simulink model "OutputToVisualizationAveragedEEG"  (R2016b)
settings: Solver=FixedStepDiscrete  StartTime=0.0  StopTime=10.0  FixedStep=sCoreParams.core.stepPeriod  RelTol=1e-3  EnableMultiTasking=on
undefined symbols (not defined in the file or in its folder): sCoreParams, sCoreParams_viz_channelInds
libraries: dspindex x3, slrtlib x2, xpcrtudplib x2, xpcutilitieslib x1, xpcobsoletelib x1
settings Model: DataTypeOverride=Double  MinMaxOverflowLogging=ForceOff  Creator=rzelmann  LastModifiedBy=Rina
settings SolverCC: EnableConcurrentExecution=on  ConcurrentTasks=on  AutoInsertRateTranBlk=on
settings DataIOCC: SaveFormat=StructureWithTime  SaveOutput=off  SignalLogging=off  DSMLogging=off  SaveTime=off
settings OptimizationCC: BlockReduction=off  DefaultParameterBehavior=Inlined  LifeSpan=inf
settings DebuggingCC: AllowSymbolicDim=off  SFUnexpectedBacktrackingDiag=warning  SFNoUnconditionalDefaultTransitionDiag=warning  SFExecutionAtInitializationDiag=none
settings HardwareCC: ProdBitPerPointer=32  ProdBitPerSizeT=32  ProdBitPerPtrDiffT=32  ProdLargestAtomicFloat=None  ProdWordSize=32  ProdLongLongMode=on  ProdHWDeviceType=Generic->32-bit x86 compatible
settings ModelReferenceCC: UpdateModelReferenceTargets=Force  ParallelModelReferenceMATLABWorkerInit=Load Top Model  ModelReferenceNumInstancesAllowed=Single  ModelReferencePassRootInputsByReference=off
settings RTWCC: SystemTargetFile=slrt.tlc  TemplateMakefile=slrt_default_tmf  Description=Simulink Real-Time  RTWCompilerOptimization=on
settings CodeAppCC: MaxIdLength=63
settings TargetCC: CodeReplacementLibrary=XPC_BLAS  ParMdlRefBuildCompliant=on  ConcurrentExecutionCompliant=on  GeneratePreprocessorConditionals=Use local settings  MatFileLogging=on  MATLABClassNameForMDSCustomization=xpcAperiodicCustomization
settings ConfigComp: CovMetricSettings=dw  CovHtmlReporting=on  CovSaveCumulativeToWorkspaceVar=on  CovSaveSingleToWorkspaceVar=on  CovExternalEMLEnable=off

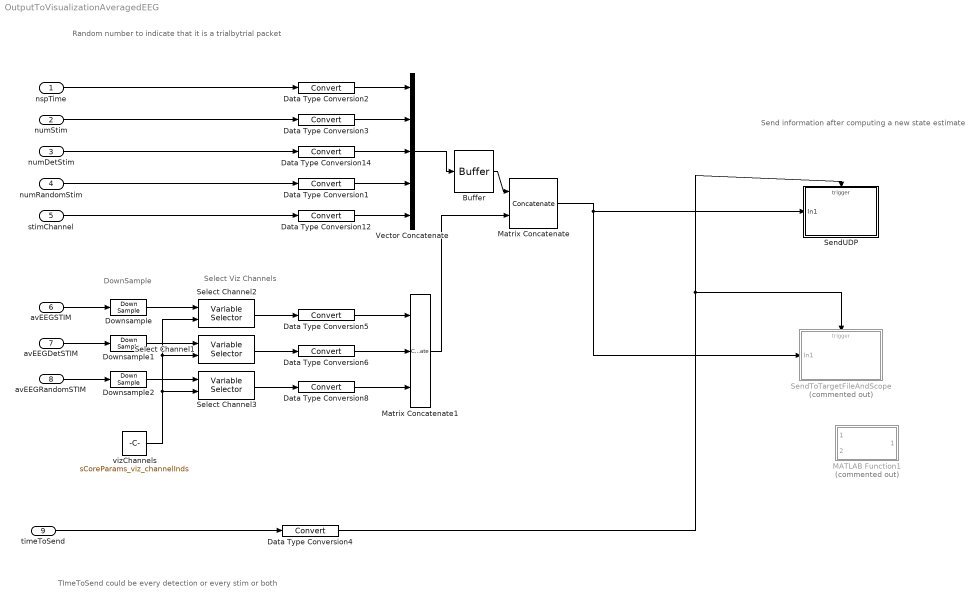
== system OutputToVisualizationAveragedEEG ==
  note: Select Viz Channels
  note: DownSample
  note: TImeToSend could be every detection or every stim or both
  note: Random number to indicate that it is a trialbytrial packet
  note: Send information after computing a new state estimate
  nspTime : Inport  PortDimensions=1  SampleTime=sCoreParams.core.stepPeriod
  numStim : Inport  Port=2  OutDataTypeStr=double  PortDimensions=1  SampleTime=sCoreParams.core.stepPeriod
  numDetStim : Inport  Port=3  OutDataTypeStr=double  PortDimensions=1  SampleTime=sCoreParams.core.stepPeriod
  numRandomStim : Inport  Port=4  PortDimensions=1  SampleTime=sCoreParams.core.stepPeriod
  stimChannel : Inport  Port=5  OutDataTypeStr=int32  PortDimensions=[1 2]  SampleTime=sCoreParams.core.stepPeriod  Interpolate=off
  avEEGSTIM : Inport  Port=6  PortDimensions=[sCoreParams.viz.DurationTriggerAvSamp sCoreParams.decoders.txDetector.nChannels]  SampleTime=sCoreParams.core.stepPeriod
  avEEGDetSTIM : Inport  Port=7  PortDimensions=[sCoreParams.viz.DurationTriggerAvSamp sCoreParams.decoders.txDetector.nChannels]  SampleTime=sCoreParams.core.stepPeriod
  avEEGRandomSTIM : Inport  Port=8  PortDimensions=[sCoreParams.viz.DurationTriggerAvSamp sCoreParams.decoders.txDetector.nChannels]  SampleTime=sCoreParams.core.stepPeriod
  timeToSend : Inport  Port=9  OutDataTypeStr=boolean  PortDimensions=1  SampleTime=sCoreParams.core.stepPeriod
  Buffer : Buffer  N=sCoreParams.write.broadcastAvEEGSamp  V=sCoreParams.write.broadcastAvEEGSamp-1  TreatMby1Signals=One channel  OutputFrames=off
  Data Type Conversion{1..6,8,12,14} (9 alike) : DataTypeConversion
  Downsample : DownSample  N=sCoreParams.write.averagedEEGDownSampling
  Downsample1 : DownSample  N=sCoreParams.write.averagedEEGDownSampling
  Downsample2 : DownSample  N=sCoreParams.write.averagedEEGDownSampling
  MATLAB Function1 : MATLAB Function  Commented=on  TreatAsAtomicUnit=on
  Matrix Concatenate : Concatenate  Mode=Multidimensional array  ConcatenateDimension=2
  Matrix Concatenate1 : Concatenate  NumInputs=3  Mode=Multidimensional array  ConcatenateDimension=2
  Select Channel1 : dspindex/Variable Selector  NumInputs=1  rowsOrCols=Columns  IdxMode=Variable  Elements=sCoreParams_decoders_txDetector_channel1  ZerOneIdxMode=One-based  errmode=Clip Index  FillMode=off  FillValues=0
  Select Channel2 : dspindex/Variable Selector  NumInputs=1  rowsOrCols=Columns  IdxMode=Variable  Elements=sCoreParams_decoders_txDetector_channel1  ZerOneIdxMode=One-based  errmode=Clip Index  FillMode=off  FillValues=0
  Select Channel3 : dspindex/Variable Selector  NumInputs=1  rowsOrCols=Columns  IdxMode=Variable  Elements=sCoreParams_decoders_txDetector_channel1  ZerOneIdxMode=One-based  errmode=Clip Index  FillMode=off  FillValues=0
  SendToTargetFileAndScope : Subsystem  Commented=on
  SendUDP : Subsystem
  Vector Concatenate : Concatenate  NumInputs=5
  vizChannels : Constant  Value=sCoreParams_viz_channelInds
  wires:
  avEEGDetSTIM/1 -> Downsample1/1
  Data Type Conversion2/1 -> Vector Concatenate/1
  Select Channel1/1 -> Data Type Conversion6/1
  Vector Concatenate/1 -> Buffer/1
  Matrix Concatenate1/1 -> Matrix Concatenate/2
  Matrix Concatenate/1 -> SendToTargetFileAndScope/1(In1), SendUDP/1(In1)
  stimChannel/1 -> Data Type Conversion12/1
  nspTime/1 -> Data Type Conversion2/1
  numStim/1 -> Data Type Conversion3/1
  avEEGSTIM/1 -> Downsample/1
  numRandomStim/1 -> Data Type Conversion1/1
  Data Type Conversion5/1 -> Matrix Concatenate1/1
  numDetStim/1 -> Data Type Conversion14/1
  Data Type Conversion14/1 -> Vector Concatenate/3
  timeToSend/1 -> Data Type Conversion4/1
  Data Type Conversion3/1 -> Vector Concatenate/2
  Data Type Conversion1/1 -> Vector Concatenate/4
  Data Type Conversion12/1 -> Vector Concatenate/5
  Data Type Conversion4/1 -> SendToTargetFileAndScope/Trigger, SendUDP/Trigger
  Data Type Conversion6/1 -> Matrix Concatenate1/2
  vizChannels/1 -> Select Channel3/2, Select Channel2/2, Select Channel1/2
  Select Channel2/1 -> Data Type Conversion5/1
  Select Channel3/1 -> Data Type Conversion8/1
  avEEGRandomSTIM/1 -> Downsample2/1
  Data Type Conversion8/1 -> Matrix Concatenate1/3
  Buffer/1 -> Matrix Concatenate/1
  Downsample/1 -> Select Channel2/1
  Downsample1/1 -> Select Channel1/1
  Downsample2/1 -> Select Channel3/1

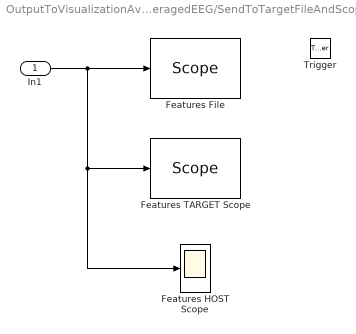
== system OutputToVisualizationAveragedEEG/SendToTargetFileAndScope ==
  In1 : Inport
  Trigger : TriggerPort  VariantControl=Variant  PortDimensions=1
  Features File : slrtlib/Displays and Logging/Scope   scopeno=2  scopetype=File  autostart=on  viewmode=Graphical redraw  formatstr='%15.6f'  grid=on  ylimits=[0,0]  nosamples=1000  noprepostsamples=-10  interleave=1  triggermode=FreeRun  triggersignal=1  trigsignalfromport=on  triggerlevel=0.0  triggerslope=Rising  triggerscope=1  triggersample=0  filename=feat_<%%%>.dat  mode=Lazy  writesize=512  autorestart=on  dynamicfilemode=on  maxwritefilesize=512*1024^2
  Features HOST Scope : Scope
  Features TARGET Scope : slrtlib/Displays and Logging/Scope   scopeno=3  scopetype=Target  autostart=on  viewmode=Graphical sliding  formatstr='%15.6f'  grid=on  ylimits=[0,0]  nosamples=1000  noprepostsamples=0  interleave=1  triggermode=FreeRun  triggersignal=1  trigsignalfromport=on  triggerlevel=0.0  triggerslope=Rising  triggerscope=1  triggersample=0  filename=data.dat  mode=Lazy  writesize=512  autorestart=off  dynamicfilemode=off  maxwritefilesize=512*1024^2
  wires:
  In1/1 -> Features HOST Scope/1, Features TARGET Scope/1, Features File/1

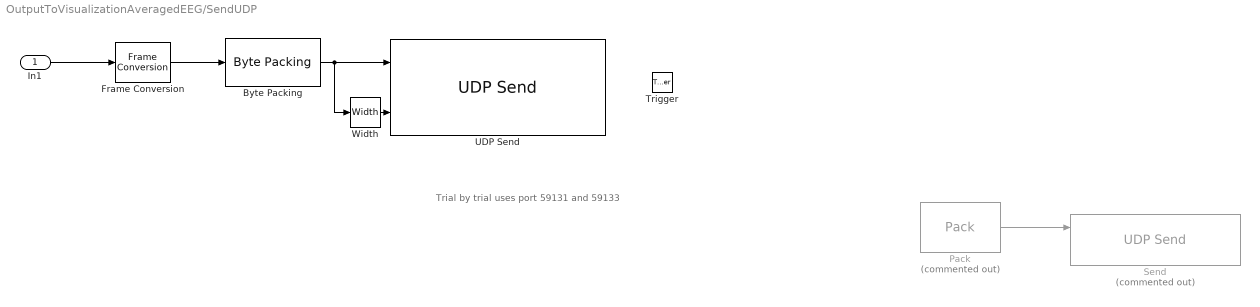
== system OutputToVisualizationAveragedEEG/SendUDP ==
  note: Trial by trial uses port 59131 and 59133
  In1 : Inport
  Trigger : TriggerPort  VariantControl=Variant  PortDimensions=1
  "Byte Packing " : xpcutilitieslib/Byte Packing   MaskPackedDataType=uint8  MaskUnpackedDataTypes={'double'}  MaskAlignment=1
  Frame Conversion : FrameConversion  InheritSamplingMode=off  OutFrame=Sample-based
  Pack : xpcobsoletelib/Utilities/Pack   Commented=on  datatypes={'double'}  byteAlign=1
  Send : xpcrtudplib/UDP Send  Commented=on  ipAddressVal=Use host-target connection  localPort=59121  toAddress=255.255.255.255  toPort=59123  sampleTime=-1
  UDP Send : xpcrtudplib/UDP Send  ipAddressVal=Use host-target connection  localPort=59141  toAddress=255.255.255.255  toPort=59143  sampleTime=-1
  Width : Width
  wires:
  "Byte Packing "/1 -> Width/1, UDP Send/1
  In1/1 -> Frame Conversion/1
  Frame Conversion/1 -> "Byte Packing "/1
  Pack/1 -> Send/1
  Width/1 -> UDP Send/2

== matlab function OutputToVisualizationAveragedEEG/MATLAB Function1 ==
  data: signalIn input; signalOut output size=[1 length(sCoreParams_viz_featureInds)]; selectCh input
function signalOut = selectChannels(signalIn,selectCh)
%#codegen
signalOut = signalIn(:,selectCh);
%signalOut = selectChannels_EML(signalIn,selectCh);
